simulink model "ArmDynamicsOnly"  (R2020a)
settings: Solver=FixedStepAuto  StartTime=0.0  StopTime=tsim  FixedStep=baseRate  MaxStep=0.0001  RelTol=1e-6  AbsTol=1e-6  EnableMultiTasking=on
values from neighbouring files (symbols this model uses):
  b0 = importdata("biases_layer_0.csv")    [Run_Initializer.m]
  b1 = importdata("biases_layer_1.csv")    [Run_Initializer.m]
  b_out = importdata("biases_output.csv")    [Run_Initializer.m]
  baseRate = 0.05    [Run_Initializer.m]
  CHASER_ABSOLUTE_POSITION = true    [Run_Initializer.m]
  drop_states_ARM = [ pi/2, pi/2, 0]    [Run_Initializer.m]
  drop_states_BLACK = [ xLength/2, yLength/2, pi]    [Run_Initializer.m]
  drop_states_BLUE = [ xLength/2, yLength/2, pi]    [Run_Initializer.m]
  drop_states_RED = [ xLength/2+0.5, yLength/2, pi]    [Run_Initializer.m]
  F_Black_X_nominal = 0.2196    [Run_Initializer.m]
  F_Black_Y_nominal = 0.2825    [Run_Initializer.m]
  F_Blue_X_nominal = 0.2196    [Run_Initializer.m]
  F_Blue_Y_nominal = 0.2825    [Run_Initializer.m]
  F_red_X_nominal = 0.2196    [Run_Initializer.m]
  F_red_Y_nominal = 0.2825    [Run_Initializer.m]
  F_thrusters_BLACK = [F_Black_X_nominal; F_Black_X_nominal;                             F_Black_Y_nominal; F_Black_Y_nominal; F_Black_X_nominal;                              F_Black_X_nominal; F_Black_Y_nominal; F_Black_Y_nominal]    [Run_Initializer.m]
  F_thrusters_BLUE = [F_Blue_X_nominal; F_Blue_X_nominal;                             F_Blue_Y_nominal; F_Blue_Y_nominal; F_Blue_X_nominal;                              F_Blue_X_nominal; F_Blue_Y_nominal; F_Blue_Y_nominal]    [Run_Initializer.m]
  F_thrusters_RED = [F_red_X_nominal; F_red_X_nominal;                             F_red_Y_nominal; F_red_Y_nominal; F_red_X_nominal;                              F_red_X_nominal; F_red_Y_nominal; F_red_Y_nominal]    [Run_Initializer.m]
  Gamma1_el = 0.12    [Run_Initializer.m]
  Gamma1_sh = 0.005    [Run_Initializer.m]
  Gamma1_wr = 0.025    [Run_Initializer.m]
  Gamma2_el = 5    [Run_Initializer.m]
  Gamma2_sh = 15    [Run_Initializer.m]
  Gamma2_wr = 5    [Run_Initializer.m]
  Gamma3_el = 10    [Run_Initializer.m]
  Gamma3_sh = 40    [Run_Initializer.m]
  Gamma3_wr = 40    [Run_Initializer.m]
  Gamma4_el = 0.039    [Run_Initializer.m]
  Gamma4_sh = 0.015    [Run_Initializer.m]
  Gamma4_wr = 0.029    [Run_Initializer.m]
  Gamma5_el = 800    [Run_Initializer.m]
  Gamma5_sh = 800    [Run_Initializer.m]
  Gamma5_wr = 800    [Run_Initializer.m]
  Gamma6_el = 0.000001    (= 1e-06)    [Run_Initializer.m]
  Gamma6_sh = 0.005    [Run_Initializer.m]
  Gamma6_wr = 0.02    [Run_Initializer.m]
  HOLD_POINT_RADIUS = 0.95    [Run_Initializer.m]
  home_states_BLACK = [ xLength/2; yLength/2; 0]    [Run_Initializer.m]
  home_states_BLUE = [ xLength/2; yLength/2; 0]    [Run_Initializer.m]
  home_states_RED = [ xLength/2+0.9; yLength/2; pi]    [Run_Initializer.m]
  init_states_BLACK = [ xLength/2; yLength/2; pi]    [Run_Initializer.m]
  init_states_BLUE = [ xLength/2; yLength/2; pi]    [Run_Initializer.m]
  init_states_RED = [ xLength/2+0.9; yLength/2; pi]    [Run_Initializer.m]
  Kd_tb = 1.0    (= 1)    [Run_Initializer.m]
  Kd_tblue = 1    [Run_Initializer.m]
  Kd_tr = 1.0    (= 1)    [Run_Initializer.m]
  Kd_xb = 8    [Run_Initializer.m]
  Kd_xblue = 8    [Run_Initializer.m]
  Kd_xr = 8    [Run_Initializer.m]
  Kd_yb = 8    [Run_Initializer.m]
  Kd_yblue = 8    [Run_Initializer.m]
  Kd_yr = 8    [Run_Initializer.m]
  Kp_tb = 0.1    [Run_Initializer.m]
  Kp_tblue = 0.1    [Run_Initializer.m]
  Kp_tr = 0.1    [Run_Initializer.m]
  Kp_xb = 2    [Run_Initializer.m]
  Kp_xblue = 2    [Run_Initializer.m]
  Kp_xr = 2    [Run_Initializer.m]
  Kp_yb = 2    [Run_Initializer.m]
  Kp_yblue = 2    [Run_Initializer.m]
  Kp_yr = 2    [Run_Initializer.m]
  MAX_BODY_ANGULAR_VELOCITY = 15*180/pi    (= 859.436692696)    [Run_Initializer.m]
  MAX_VELOCITY = 0.1    [Run_Initializer.m]
  noise_variance_BLACK = 0    [Run_Initializer.m]
  noise_variance_BLUE = 0    [Run_Initializer.m]
  noise_variance_RED = 0    [Run_Initializer.m]
  Phase0_End = Phase0_Duration    (= 10)    [Run_Initializer.m]
  Phase1_End = Phase0_Duration + Phase1_Duration    (= 15)    [Run_Initializer.m]
  Phase2_End = Phase0_Duration + Phase1_Duration +                                   Phase2_Duration    (= 45)    [Run_Initializer.m]
  Phase3_End = Phase0_Duration + Phase1_Duration +                                   Phase2_Duration + Phase3_Duration    (= 560)    [Run_Initializer.m]
  Phase3_SubPhase1_End = Phase2_End + Phase3_SubPhase1_Duration    (= 105)    [Run_Initializer.m]
  Phase3_SubPhase2_End = Phase2_End + Phase3_SubPhase1_Duration +                                   Phase3_SubPhase2_Duration    (= 210)    [Run_Initializer.m]
  Phase3_SubPhase3_End = Phase2_End + Phase3_SubPhase1_Duration +                                   Phase3_SubPhase2_Duration +                                  Phase3_SubPhase3_Duration    (= 240)    [Run_Initializer.m]
  Phase3_SubPhase4_End = Phase2_End + Phase3_SubPhase1_Duration +                                   Phase3_SubPhase2_Duration +                                  Phase3_SubPhase3_Duration +                                  Phase3_SubPhase4_Duration    [Run_Initializer.m]
  Phase4_End = Phase0_Duration + Phase1_Duration +                                   Phase2_Duration + Phase3_Duration +                                   Phase4_Duration    (= 680)    [Run_Initializer.m]
  Phase5_End = Phase0_Duration + Phase1_Duration +                                   Phase2_Duration + Phase3_Duration +                                   Phase4_Duration + Phase5_Duration    (= 700)    [Run_Initializer.m]
  relevant_half_range = (upper_state_bound - lower_state_bound)/2    [Run_Initializer.m]
  relevant_state_mean = (lower_state_bound + upper_state_bound)/2    [Run_Initializer.m]
  thruster_dist2CG_BLACK = [72.80;-65.20;61.75;-79.75;65.20;-65.20;74.25;-54.75]    [Run_Initializer.m]
  thruster_dist2CG_BLUE = [83.10;-54.90;71.50;-70.00;54.90;-75.50;64.50;-64.50]    [Run_Initializer.m]
  thruster_dist2CG_RED = [69.38;-56.62;50.01;-81.49;61.12;-68.38;78.99;-52.01]    [Run_Initializer.m]
  w0 = importdata("weights_layer_0.csv")    [Run_Initializer.m]
  w1 = importdata("weights_layer_1.csv")    [Run_Initializer.m]
  w_out = importdata("weights_output.csv")    [Run_Initializer.m]
  xLength = 3.51155    [Run_Initializer.m]
  yLength = 2.41935    [Run_Initializer.m]
undefined symbols (not defined in the file or in its folder): DiscIntNeverNeededParam, model_param, platformSelection, serverRate, simMode
libraries: dspstat3 x18, simulink x11, raspberrypiBasiclib x9, dspsigops x9, embdlinuxlib x7, MainLibrary x4, mspfiltlib x3, dsparch4 x3, etargetslib x1, sensehatlib x1
(part 12 of 14)

== matlab function ArmDynamicsOnly/Calculate Thruster ON//OFF/MATLAB Function7 ==
  data: H output; thruster_dist2CG_RED parameter; F_thrusters_RED parameter
function H = MakeH(thruster_dist2CG_RED,F_thrusters_RED)

Vec1 = [ -1
         -1
          0 
          0
          1
          1
          0
          0 ];
      
Vec2 = [  0
          0
          1
          1
          0
          0
         -1
         -1 ];
     
Vec3 = thruster_dist2CG_RED./1000;

Mat1 = [Vec1, Vec2, Vec3]';

Mat2 = diag((F_thrusters_RED./2));

H    = Mat1*Mat2;

end

== matlab function ArmDynamicsOnly/Calculate Thruster ON//OFF/MATLAB Function8 ==
  data: H output; thruster_dist2CG_RED parameter; F_red_X_nominal parameter; theta_1 input; theta_2 input; theta_3 input; model_param parameter; thrust_decay_factor input; F_red_Y_nominal parameter
function H   = MakeH(thruster_dist2CG_RED,F_red_X_nominal, theta_1, theta_2, theta_3, model_param, thrust_decay_factor, F_red_Y_nominal)


m0  = model_param(1);          
phi = model_param(7);
b0  = model_param(8);
a1  = model_param(9);
b1  = model_param(10);              
a2  = model_param(11);                
b2  = model_param(12);               
a3  = model_param(13);                         
m1  = model_param(15);
m2  = model_param(16);
m3  = model_param(17);

link1_com_x = b0*cos(phi) + a1*cos(pi/2 + theta_1);
link1_com_y = b0*sin(phi) + a1*sin(pi/2 + theta_1);

link2_com_x = link1_com_x + b1*cos(pi/2 + theta_1) + a2*cos(pi/2 + theta_1 + theta_2);
link2_com_y = link1_com_y + b1*sin(pi/2 + theta_1) + a2*sin(pi/2 + theta_1 + theta_2);

link3_com_x = link2_com_x + b2*cos(pi/2 + theta_1 + theta_2) + a3*cos(pi/2 + theta_1 + theta_2 + theta_3);
link3_com_y = link2_com_y + b2*sin(pi/2 + theta_1 + theta_2) + a3*sin(pi/2 + theta_1 + theta_2 + theta_3);

delta_com_due_to_arm_x = (m1*link1_com_x + m2*link2_com_x + m3*link3_com_x)/(m0 + m1 + m2 + m3)*1000; % [mm]
delta_com_due_to_arm_y = (m1*link1_com_y + m2*link2_com_y + m3*link3_com_y)/(m0 + m1 + m2 + m3)*1000; % [mm]

adjusted_thruster_dist2CG_RED = [thruster_dist2CG_RED(1)-delta_com_due_to_arm_y;
                                 thruster_dist2CG_RED(2)-delta_com_due_to_arm_y;
                                 thruster_dist2CG_RED(3)-delta_com_due_to_arm_x;
                                 thruster_dist2CG_RED(4)-delta_com_due_to_arm_x;
                                 thruster_dist2CG_RED(5)+delta_com_due_to_arm_y;
                                 thruster_dist2CG_RED(6)+delta_com_due_to_arm_y;
                                 thruster_dist2CG_RED(7)+delta_com_due_to_arm_x;
                                 thruster_dist2CG_RED(8)+delta_com_due_to_arm_x];
                                 


Vec1 = [ -1
         -1
          0 
          0
          1
          1
          0
          0 ];
      
Vec2 = [  0
          0
          1
          1
          0
          0
         -1
         -1 ];
     
Vec3 = adjusted_thruster_dist2CG_RED./1000;

Mat1 = [Vec1, Vec2, Vec3]';

F_thrusters_RED = [F_red_X_nominal*thrust_decay_factor; F_red_X_nominal*thrust_decay_factor; F_red_Y_nominal*thrust_decay_factor; F_red_Y_nominal*thrust_decay_factor; F_red_X_nominal*thrust_decay_factor; F_red_X_nominal*thrust_decay_factor; F_red_Y_nominal*thrust_decay_factor; F_red_Y_nominal*thrust_decay_factor];

Mat2 = diag((F_thrusters_RED));

H    = Mat1*Mat2;

end

== matlab function ArmDynamicsOnly/Calculate Thruster ON//OFF/MATLAB Function9 ==
  data: thrust_decay_factor output; PWMs input; thruster_count_threshold parameter; count output
function [thrust_decay_factor, count]  = check_thrust_decay(PWMs,thruster_count_threshold)

% normalize PWMs
if max(PWMs) > 1
    PWMs = PWMs/max(PWMs);
end

count = sum(PWMs > thruster_count_threshold);

positives_only = max(PWMs,0);
sum_of_duty_cycles = sum(positives_only);

average_duty_cycle_per_thruster = sum_of_duty_cycles/count;

% Look up the thrust decay for this average duty cycle
if (average_duty_cycle_per_thruster < 0.3) || (count == 0)
    thrust_decay_factor = 1;
else
    thrust_decay_factor = max(0.6 - 2*average_duty_cycle_per_thruster + 1, 0.5);   
end

== matlab function ArmDynamicsOnly/Calculate Thruster ON//OFF/Rotate Forces to Inertial1/Create Rotation Matrix ==
  data: Rz input; C_Ib output
function C_Ib = RotateFrame(Rz)

C_bI = [  cos(Rz) sin(Rz)
         -sin(Rz) cos(Rz) ];

C_Ib = inv(C_bI);

end

== matlab function ArmDynamicsOnly/Rotate Forces to Body/Create Rotation Matrix ==
  data: Rz input; C_bI output
function C_bI = RotateFrame(Rz)

C_bI = [  cos(Rz) sin(Rz)
         -sin(Rz) cos(Rz) ];

end

== matlab function ArmDynamicsOnly/Phase #5: Hold Home/Change RED Behavior/Hough Control/MATLAB Function2 ==
  data: Oy output; z input; Ox output
function [Oy, Ox]   = C3( z )
%C3 gives the rotation matrix about the z-axis for an angle 'z'
%   z - the angle about the z-axis which you rotate
%   A - the rotation matrix

Ox = [cos(z) sin(z); -sin(z) cos(z)]*[1;0];
Oy = [cos(z) sin(z); -sin(z) cos(z)]*[0;1];
end

== matlab function ArmDynamicsOnly/Phase #5: Hold Home/Change RED Behavior/Hough Control/MATLAB Function3 ==
  data: z input; Ox output
function Ox    = C3( z )
%C3 gives the rotation matrix about the z-axis for an angle 'z'
%   z - the angle about the z-axis which you rotate
%   A - the rotation matrix

Ox = [cos(z) sin(z); -sin(z) cos(z)]*[1;0];
end

== matlab function ArmDynamicsOnly/Phase #2: Move to Initial Position/Change BLACK Behavior/Hough Control/MATLAB Function3 ==
  data: z input; Ox output
function Ox    = C3( z )
%C3 gives the rotation matrix about the z-axis for an angle 'z'
%   z - the angle about the z-axis which you rotate
%   A - the rotation matrix

Ox = [cos(z) sin(z); -sin(z) cos(z)]*[1;0];
end

== matlab function ArmDynamicsOnly/Phase #5: Hold Home/Change RED Behavior/Hough Control/MATLAB Function4 ==
  data: Oy input; e_out output; e_in input
function e_out = fcn(Oy, e_in)

a = sign(Oy'*e_in);
e_out = -a*norm(e_in);

== matlab function ArmDynamicsOnly/From Force//Torque to PWM Signal/Change RED Behavior/Calculate Thruster ON//OFF/MATLAB Function10 ==
  data: H output; thruster_dist2CG_RED parameter; F_red_X_nominal parameter; theta_1 input; theta_2 input; theta_3 input; model_param parameter; thrust_decay_factor input; F_red_Y_nominal parameter
function H   = MakeHWithArmAndDecay(thruster_dist2CG_RED,F_red_X_nominal, theta_1, theta_2, theta_3, model_param, thrust_decay_factor, F_red_Y_nominal)

m0  = model_param(1);          
phi = model_param(7);
b0  = model_param(8);
a1  = model_param(9);
b1  = model_param(10);              
a2  = model_param(11);                
b2  = model_param(12);               
a3  = model_param(13);                         
m1  = model_param(15);
m2  = model_param(16);
m3  = model_param(17);

link1_com_x = b0*cos(phi) + a1*cos(pi/2 + theta_1);
link1_com_y = b0*sin(phi) + a1*sin(pi/2 + theta_1);

link2_com_x = link1_com_x + b1*cos(pi/2 + theta_1) + a2*cos(pi/2 + theta_1 + theta_2);
link2_com_y = link1_com_y + b1*sin(pi/2 + theta_1) + a2*sin(pi/2 + theta_1 + theta_2);

link3_com_x = link2_com_x + b2*cos(pi/2 + theta_1 + theta_2) + a3*cos(pi/2 + theta_1 + theta_2 + theta_3);
link3_com_y = link2_com_y + b2*sin(pi/2 + theta_1 + theta_2) + a3*sin(pi/2 + theta_1 + theta_2 + theta_3);

delta_com_due_to_arm_x = (m1*link1_com_x + m2*link2_com_x + m3*link3_com_x)/(m0 + m1 + m2 + m3)*1000; % [mm]
delta_com_due_to_arm_y = (m1*link1_com_y + m2*link2_com_y + m3*link3_com_y)/(m0 + m1 + m2 + m3)*1000; % [mm]

adjusted_thruster_dist2CG_RED = [thruster_dist2CG_RED(1)-delta_com_due_to_arm_y;
                                 thruster_dist2CG_RED(2)-delta_com_due_to_arm_y;
                                 thruster_dist2CG_RED(3)-delta_com_due_to_arm_x;
                                 thruster_dist2CG_RED(4)-delta_com_due_to_arm_x;
                                 thruster_dist2CG_RED(5)+delta_com_due_to_arm_y;
                                 thruster_dist2CG_RED(6)+delta_com_due_to_arm_y;
                                 thruster_dist2CG_RED(7)+delta_com_due_to_arm_x;
                                 thruster_dist2CG_RED(8)+delta_com_due_to_arm_x];
                                 


Vec1 = [ -1
         -1
          0 
          0
          1
          1
          0
          0 ];
      
Vec2 = [  0
          0
          1
          1
          0
          0
         -1
         -1 ];
     
Vec3 = adjusted_thruster_dist2CG_RED./1000;

Mat1 = [Vec1, Vec2, Vec3]';

F_thrusters_RED = [F_red_X_nominal*thrust_decay_factor; F_red_X_nominal*thrust_decay_factor; F_red_Y_nominal*thrust_decay_factor; F_red_Y_nominal*thrust_decay_factor; F_red_X_nominal*thrust_decay_factor; F_red_X_nominal*thrust_decay_factor; F_red_Y_nominal*thrust_decay_factor; F_red_Y_nominal*thrust_decay_factor];

Mat2 = diag((F_thrusters_RED./2));

H    = Mat1*Mat2;

end

== matlab function ArmDynamicsOnly/From Force//Torque to PWM Signal/Change RED Behavior/Calculate Thruster ON//OFF/MATLAB Function3 ==
  data: H output; thruster_dist2CG_RED parameter; F_thrusters_RED parameter; theta_1 input; theta_2 input; theta_3 input; model_param parameter
function H   = MakeHWithArm(thruster_dist2CG_RED,F_thrusters_RED, theta_1, theta_2, theta_3, model_param)

m0  = model_param(1);          
phi = model_param(7);
b0  = model_param(8);
a1  = model_param(9);
b1  = model_param(10);              
a2  = model_param(11);                
b2  = model_param(12);               
a3  = model_param(13);                         
m1  = model_param(15);
m2  = model_param(16);
m3  = model_param(17);

link1_com_x = b0*cos(phi) + a1*cos(pi/2 + theta_1);
link1_com_y = b0*sin(phi) + a1*sin(pi/2 + theta_1);

link2_com_x = link1_com_x + b1*cos(pi/2 + theta_1) + a2*cos(pi/2 + theta_1 + theta_2);
link2_com_y = link1_com_y + b1*sin(pi/2 + theta_1) + a2*sin(pi/2 + theta_1 + theta_2);

link3_com_x = link2_com_x + b2*cos(pi/2 + theta_1 + theta_2) + a3*cos(pi/2 + theta_1 + theta_2 + theta_3);
link3_com_y = link2_com_y + b2*sin(pi/2 + theta_1 + theta_2) + a3*sin(pi/2 + theta_1 + theta_2 + theta_3);

delta_com_due_to_arm_x = (m1*link1_com_x + m2*link2_com_x + m3*link3_com_x)/(m0 + m1 + m2 + m3)*1000; % [mm]
delta_com_due_to_arm_y = (m1*link1_com_y + m2*link2_com_y + m3*link3_com_y)/(m0 + m1 + m2 + m3)*1000; % [mm]

adjusted_thruster_dist2CG_RED = [thruster_dist2CG_RED(1)-delta_com_due_to_arm_y;
                                 thruster_dist2CG_RED(2)-delta_com_due_to_arm_y;
                                 thruster_dist2CG_RED(3)-delta_com_due_to_arm_x;
                                 thruster_dist2CG_RED(4)-delta_com_due_to_arm_x;
                                 thruster_dist2CG_RED(5)+delta_com_due_to_arm_y;
                                 thruster_dist2CG_RED(6)+delta_com_due_to_arm_y;
                                 thruster_dist2CG_RED(7)+delta_com_due_to_arm_x;
                                 thruster_dist2CG_RED(8)+delta_com_due_to_arm_x];
                                 


Vec1 = [ -1
         -1
          0 
          0
          1
          1
          0
          0 ];
      
Vec2 = [  0
          0
          1
          1
          0
          0
         -1
         -1 ];
     
Vec3 = adjusted_thruster_dist2CG_RED./1000;

Mat1 = [Vec1, Vec2, Vec3]';

Mat2 = diag((F_thrusters_RED./2));

H    = Mat1*Mat2;

end

== matlab function ArmDynamicsOnly/From Force//Torque to PWM Signal/Change RED Behavior/Calculate Thruster ON//OFF/MATLAB Function4 ==
  data: H output; thruster_dist2CG_RED parameter; F_thrusters_RED parameter
function H = MakeH(thruster_dist2CG_RED,F_thrusters_RED)

Vec1 = [ -1
         -1
          0 
          0
          1
          1
          0
          0 ];
      
Vec2 = [  0
          0
          1
          1
          0
          0
         -1
         -1 ];
     
Vec3 = thruster_dist2CG_RED./1000;

Mat1 = [Vec1, Vec2, Vec3]';

Mat2 = diag((F_thrusters_RED));

H    = Mat1*Mat2;

end

== matlab function ArmDynamicsOnly/From Force//Torque to PWM Signal/Change RED Behavior/Calculate Thruster ON//OFF/MATLAB Function6 ==
  data: ThrustPer_Final output; ThrustPer input
function ThrustPer_Final  = ThrusterSat(ThrustPer)

ValveTime       = 0.007;
TControl        = 0.1;
ThrustPer_Final = zeros(8,1);

if max(ThrustPer) > 1
    ThrustPer_Sat = ThrustPer/max(ThrustPer);
else
    ThrustPer_Sat = ThrustPer;
end

for i = 1:8
    if ThrustPer_Sat(i) > ValveTime/TControl 
        ThrustPer_Final(i) = ThrustPer_Sat(i);
    else
        ThrustPer_Final(i) = 0;
    end
end
   

end

== matlab function ArmDynamicsOnly/From Force//Torque to PWM Signal/Change RED Behavior/Calculate Thruster ON//OFF/MATLAB Function7 ==
  data: H output; thruster_dist2CG_RED parameter; F_thrusters_RED parameter
function H = MakeH(thruster_dist2CG_RED,F_thrusters_RED)

Vec1 = [ -1
         -1
          0 
          0
          1
          1
          0
          0 ];
      
Vec2 = [  0
          0
          1
          1
          0
          0
         -1
         -1 ];
     
Vec3 = thruster_dist2CG_RED./1000;

Mat1 = [Vec1, Vec2, Vec3]';

Mat2 = diag((F_thrusters_RED./2));

H    = Mat1*Mat2;

end

== matlab function ArmDynamicsOnly/From Force//Torque to PWM Signal/Change RED Behavior/Calculate Thruster ON//OFF/MATLAB Function8 ==
  data: H output; thruster_dist2CG_RED parameter; F_red_X_nominal parameter; theta_1 input; theta_2 input; theta_3 input; model_param parameter; thrust_decay_factor input; F_red_Y_nominal parameter
function H   = MakeH(thruster_dist2CG_RED,F_red_X_nominal, theta_1, theta_2, theta_3, model_param, thrust_decay_factor, F_red_Y_nominal)


m0  = model_param(1);          
phi = model_param(7);
b0  = model_param(8);
a1  = model_param(9);
b1  = model_param(10);              
a2  = model_param(11);                
b2  = model_param(12);               
a3  = model_param(13);                         
m1  = model_param(15);
m2  = model_param(16);
m3  = model_param(17);

link1_com_x = b0*cos(phi) + a1*cos(pi/2 + theta_1);
link1_com_y = b0*sin(phi) + a1*sin(pi/2 + theta_1);

link2_com_x = link1_com_x + b1*cos(pi/2 + theta_1) + a2*cos(pi/2 + theta_1 + theta_2);
link2_com_y = link1_com_y + b1*sin(pi/2 + theta_1) + a2*sin(pi/2 + theta_1 + theta_2);

link3_com_x = link2_com_x + b2*cos(pi/2 + theta_1 + theta_2) + a3*cos(pi/2 + theta_1 + theta_2 + theta_3);
link3_com_y = link2_com_y + b2*sin(pi/2 + theta_1 + theta_2) + a3*sin(pi/2 + theta_1 + theta_2 + theta_3);

delta_com_due_to_arm_x = (m1*link1_com_x + m2*link2_com_x + m3*link3_com_x)/(m0 + m1 + m2 + m3)*1000; % [mm]
delta_com_due_to_arm_y = (m1*link1_com_y + m2*link2_com_y + m3*link3_com_y)/(m0 + m1 + m2 + m3)*1000; % [mm]

adjusted_thruster_dist2CG_RED = [thruster_dist2CG_RED(1)-delta_com_due_to_arm_y;
                                 thruster_dist2CG_RED(2)-delta_com_due_to_arm_y;
                                 thruster_dist2CG_RED(3)-delta_com_due_to_arm_x;
                                 thruster_dist2CG_RED(4)-delta_com_due_to_arm_x;
                                 thruster_dist2CG_RED(5)+delta_com_due_to_arm_y;
                                 thruster_dist2CG_RED(6)+delta_com_due_to_arm_y;
                                 thruster_dist2CG_RED(7)+delta_com_due_to_arm_x;
                                 thruster_dist2CG_RED(8)+delta_com_due_to_arm_x];
                                 


Vec1 = [ -1
         -1
          0 
          0
          1
          1
          0
          0 ];
      
Vec2 = [  0
          0
          1
          1
          0
          0
         -1
         -1 ];
     
Vec3 = adjusted_thruster_dist2CG_RED./1000;

Mat1 = [Vec1, Vec2, Vec3]';

F_thrusters_RED = [F_red_X_nominal*thrust_decay_factor; F_red_X_nominal*thrust_decay_factor; F_red_Y_nominal*thrust_decay_factor; F_red_Y_nominal*thrust_decay_factor; F_red_X_nominal*thrust_decay_factor; F_red_X_nominal*thrust_decay_factor; F_red_Y_nominal*thrust_decay_factor; F_red_Y_nominal*thrust_decay_factor];

Mat2 = diag((F_thrusters_RED));

H    = Mat1*Mat2;

end

== matlab function ArmDynamicsOnly/Phase #2: Move to Initial Position/Change BLACK Behavior/Hough Control/MATLAB Function4 ==
  data: Oy input; e_out output; e_in input
function e_out = fcn(Oy, e_in)

a = sign(Oy'*e_in);
e_out = -a*norm(e_in);

== matlab function ArmDynamicsOnly/From Force//Torque to PWM Signal/Change RED Behavior/Calculate Thruster ON//OFF/MATLAB Function9 ==
  data: thrust_decay_factor output; PWMs input; thruster_count_threshold parameter; count output
function [thrust_decay_factor, count]  = check_thrust_decay(PWMs,thruster_count_threshold)

% normalize PWMs
if max(PWMs) > 1
    PWMs = PWMs/max(PWMs);
end

count = sum(PWMs > thruster_count_threshold);

positives_only = max(PWMs,0);
sum_of_duty_cycles = sum(positives_only);

average_duty_cycle_per_thruster = sum_of_duty_cycles/count;

% Look up the thrust decay for this average duty cycle
if (average_duty_cycle_per_thruster < 0.3) || (count == 0)
    thrust_decay_factor = 1;
else
    thrust_decay_factor = max(0.6 - 2*average_duty_cycle_per_thruster + 1, 0.5);   
end

== matlab function ArmDynamicsOnly/From Force//Torque to PWM Signal/Change RED Behavior/Calculate Thruster ON//OFF/Rotate Forces to Inertial1/Create Rotation Matrix ==
  data: Rz input; C_Ib output
function C_Ib = RotateFrame(Rz)

C_bI = [  cos(Rz) sin(Rz)
         -sin(Rz) cos(Rz) ];

C_Ib = inv(C_bI);

end

== matlab function ArmDynamicsOnly/From Force//Torque to PWM Signal/Change BLACK Behavior/Calculate Thruster ON//OFF/MATLAB Function ==
  data: H output; thruster_dist2CG_BLACK parameter; F_thrusters_BLACK parameter
function H = MakeH(thruster_dist2CG_BLACK,F_thrusters_BLACK)

Vec1 = [ -1
         -1
          0 
          0
          1
          1
          0
          0 ];
      
Vec2 = [  0
          0
          1
          1
          0
          0
         -1
         -1 ];
     
Vec3 = thruster_dist2CG_BLACK./1000;

Mat1 = [Vec1, Vec2, Vec3]';

Mat2 = diag((F_thrusters_BLACK./2));

H    = Mat1*Mat2;

end

== matlab function ArmDynamicsOnly/Phase #3: Experiment/Change BLACK Behavior/Sub-Phase #4/BLACK_RzD/Wrap1/MATLAB Function ==
  data: u input; wrappedAngle output
function wrappedAngle = wrapAngle(u)

wrappedAngle = atan2(sin(u),cos(u));

end

== matlab function ArmDynamicsOnly/Phase #3: Experiment/Change BLACK Behavior/Sub-Phase #2 /BLACK_RzD1/Wrap1/MATLAB Function ==
  data: u input; wrappedAngle output
function wrappedAngle = wrapAngle(u)

wrappedAngle = atan2(sin(u),cos(u));

end

== matlab function ArmDynamicsOnly/From Force//Torque to PWM Signal/Change BLACK Behavior/Calculate Thruster ON//OFF/MATLAB Function1 ==
  data: H output; thruster_dist2CG_BLACK parameter; F_thrusters_BLACK parameter
function H = MakeH(thruster_dist2CG_BLACK,F_thrusters_BLACK)

Vec1 = [ -1
         -1
          0 
          0
          1
          1
          0
          0 ];
      
Vec2 = [  0
          0
          1
          1
          0
          0
         -1
         -1 ];
     
Vec3 = thruster_dist2CG_BLACK./1000;

Mat1 = [Vec1, Vec2, Vec3]';

Mat2 = diag((F_thrusters_BLACK));

H    = Mat1*Mat2;

end

== matlab function ArmDynamicsOnly/From Force//Torque to PWM Signal/Change BLACK Behavior/Calculate Thruster ON//OFF/MATLAB Function2 ==
  data: ThrustPer_Final output; ThrustPer input
function ThrustPer_Final  = ThrusterSat(ThrustPer)

ValveTime       = 0.007;
TControl        = 0.1;
ThrustPer_Final = zeros(8,1);

if max(ThrustPer) > 1
    ThrustPer_Sat = ThrustPer/max(ThrustPer);
else
    ThrustPer_Sat = ThrustPer;
end

for i = 1:8
    if ThrustPer_Sat(i) > ValveTime/TControl 
        ThrustPer_Final(i) = ThrustPer_Sat(i);
    else
        ThrustPer_Final(i) = 0;
    end
end
   

end

== matlab function ArmDynamicsOnly/From Force//Torque to PWM Signal/Change BLACK Behavior/Calculate Thruster ON//OFF/Rotate Forces to Inertial/Create Rotation Matrix ==
  data: Rz input; C_Ib output
function C_Ib = RotateFrame(Rz)

C_bI = [  cos(Rz) sin(Rz)
         -sin(Rz) cos(Rz) ];

C_Ib = inv(C_bI);

end

== matlab function ArmDynamicsOnly/From Force//Torque to PWM Signal/Change BLACK Behavior/Rotate Forces to Body/Create Rotation Matrix ==
  data: Rz input; C_bI output
function C_bI = RotateFrame(Rz)

C_bI = [  cos(Rz) sin(Rz)
         -sin(Rz) cos(Rz) ];

end

== matlab function ArmDynamicsOnly/Phase #3: Experiment/Change RED Behavior/Sub-Phase #2 /Hough Control/MATLAB Function2 ==
  data: Oy output; z input; Ox output
function [Oy, Ox]   = C3( z )
%C3 gives the rotation matrix about the z-axis for an angle 'z'
%   z - the angle about the z-axis which you rotate
%   A - the rotation matrix

Ox = [cos(z) sin(z); -sin(z) cos(z)]*[1;0];
Oy = [cos(z) sin(z); -sin(z) cos(z)]*[0;1];
end

== matlab function ArmDynamicsOnly/Phase #3: Experiment/Change RED Behavior/Sub-Phase #3 /Hough Control/MATLAB Function2 ==
  data: Oy output; z input; Ox output
function [Oy, Ox]   = C3( z )
%C3 gives the rotation matrix about the z-axis for an angle 'z'
%   z - the angle about the z-axis which you rotate
%   A - the rotation matrix

Ox = [cos(z) sin(z); -sin(z) cos(z)]*[1;0];
Oy = [cos(z) sin(z); -sin(z) cos(z)]*[0;1];
end

== matlab function ArmDynamicsOnly/Phase #3: Experiment/Change RED Behavior/Sub-Phase #4/calculate_mass_matrix ==
  data: M output
function M  = generate_M()
  
    m0                 = 13.80;     % RED Mass
    I0                = 0.242150;      % RED Inertia;
   


    M = [m0 0 0
         0 m0 0
         0 0 I0];

end
% Artificially setting M_31 and M_32 to zero, such that the feedforward
% controller does not think a torque needs to be applied to the base to
% counteract the torque needed to maintain the angular acceleration of the
% links when the base has a linear acceleration. No torque is applied to keep the links at their linear
% acceleration because friction does this for us.

% The original matrix
% M = reshape([t17,0.0,t30,-t86-t87-t88,-t88-t13.*t28,-t88,...
%     0.0,t17,t33,-t89-t90-t91,-t91-t24.*t28,-t91,...
%     t30,t33,...
%     I0+I1+I2+I3+t46+t51+t57+t64+t65+t66+t67+t68+t70+t71+t72+t74+t75+t76+t77+t59.*(a1.*b0.*m1.*2.0+a1.*b0.*m2.*2.0+a1.*b0.*m3.*2.0+b0.*b1.*m2.*2.0+b0.*b1.*m3.*2.0)+m1.*t36+m2.*t36+m3.*t36-t61.*(a2.*b0.*m2.*2.0+a2.*b0.*m3.*2.0+b0.*b2.*m3.*2.0)-a3.*b0.*m3.*t63.*2.0,t99,I2+I3+t51+t67+t68+t70+t74+t77+t85+t107-t112-t113,I3+t70+t85+t111-t113,-t7.*t8-t13.*t14-a3.*m3.*t16,    -t8.*t23-t14.*t24-a3.*m3.*t25,t99,I1+I2+I3+t46+t51+t57+t64+t65+t66+t67+t68+t70+t71+t72+t74+t75+t76+t77,t114,t115,-t13.*t28-a3.*m3.*t16,-t24.*t28-a3.*m3.*t25,I2+I3+t51+t67+t68+t70+t74+t77+t85+t107-t61.*t81-a3.*b0.*m3.*t63,t114,I2+I3+t51+t67+t68+t70+t74+t77,t116,-a3.*m3.*t16,-a3.*m3.*t25,I3+t70+t85+t111-a3.*b0.*m3.*t63,t115,t116,I3+t70],[6,6]);

== matlab function ArmDynamicsOnly/Phase #3: Experiment/Change RED Behavior/Sub-Phase #4/RED+ARM/Transpose Jacobian Controller/Arm Controller/MATLAB Function ==
  data: dx input; dxd input; dxi input; TAU output; qdot input; Jt input
function TAU  = fcn(dx, dxd, dxi, qdot, Jt)
%#codegen

Kp = [1500 0 0
      0    1500 0
      0    0    1500];
Kv = [50 0 0
      0    50 0
      0    0    50];    
Ki = [200 0 0
      0    200 0
      0    0    200]; 
% Source: http://ieeexplore.ieee.org.proxy.library.carleton.ca/stamp/stamp.jsp?tp=&arnumber=34766
q1_d   = qdot(1);
q2_d   = qdot(2);
q3_d   = qdot(3);

% Control Law
TAU = Kp*Jt*dx' + Kv*Jt*dxd' + Ki*Jt*dxi';% + Kv*[ q1_d q2_d q3_d];
                   

end

== matlab function ArmDynamicsOnly/Simulate Plant Dynamics/RED and ARM Dynamics/RED Only/RED Dynamics/Sample and Hold Data to Match PhaseSpace (RED)/MATLAB Function ==
  data: TIME input; y output; SERVER input
function y = fcn(TIME, SERVER)

if mod(TIME,SERVER) == 0
    y = 1;
else
    y = 0;
end

== matlab function ArmDynamicsOnly/Simulate Plant Dynamics/BLACK Dynamics/Sample and Hold Data to Match PhaseSpace (BLACK)/MATLAB Function ==
  data: TIME input; y output; SERVER input
function y = fcn(TIME, SERVER)

if mod(TIME,SERVER) == 0
    y = 1;
else
    y = 0;
end

== matlab function ArmDynamicsOnly/From Force//Torque to PWM Signal/Change RED Behavior/Rotate Forces to Body/Create Rotation Matrix ==
  data: Rz input; C_bI output
function C_bI = RotateFrame(Rz)

C_bI = [  cos(Rz) sin(Rz)
         -sin(Rz) cos(Rz) ];

end

== matlab function ArmDynamicsOnly/Phase #2: Move to Initial Position/Change RED Behavior/Hough Control/MATLAB Function2 ==
  data: Oy output; z input; Ox output
function [Oy, Ox]   = C3( z )
%C3 gives the rotation matrix about the z-axis for an angle 'z'
%   z - the angle about the z-axis which you rotate
%   A - the rotation matrix

Ox = [cos(z) sin(z); -sin(z) cos(z)]*[1;0];
Oy = [cos(z) sin(z); -sin(z) cos(z)]*[0;1];
end

== matlab function ArmDynamicsOnly/Phase #2: Move to Initial Position/Change RED Behavior/Hough Control/MATLAB Function3 ==
  data: z input; Ox output
function Ox    = C3( z )
%C3 gives the rotation matrix about the z-axis for an angle 'z'
%   z - the angle about the z-axis which you rotate
%   A - the rotation matrix

Ox = [cos(z) sin(z); -sin(z) cos(z)]*[1;0];
end

== matlab function ArmDynamicsOnly/Phase #2: Move to Initial Position/Change RED Behavior/Hough Control/MATLAB Function4 ==
  data: Oy input; e_out output; e_in input
function e_out = fcn(Oy, e_in)

a = sign(Oy'*e_in);
e_out = -a*norm(e_in);

== matlab function ArmDynamicsOnly/Phase #3: Experiment/Change BLACK Behavior/Sub-Phase #2 /Hough Control/MATLAB Function2 ==
  data: Oy output; z input; Ox output
function [Oy, Ox]   = C3( z )
%C3 gives the rotation matrix about the z-axis for an angle 'z'
%   z - the angle about the z-axis which you rotate
%   A - the rotation matrix

Ox = [cos(z) sin(z); -sin(z) cos(z)]*[1;0];
Oy = [cos(z) sin(z); -sin(z) cos(z)]*[0;1];
end

== matlab function ArmDynamicsOnly/Phase #4: Return Home/Change BLACK Behavior/Hough Control/MATLAB Function2 ==
  data: Oy output; z input; Ox output
function [Oy, Ox]   = C3( z )
%C3 gives the rotation matrix about the z-axis for an angle 'z'
%   z - the angle about the z-axis which you rotate
%   A - the rotation matrix

Ox = [cos(z) sin(z); -sin(z) cos(z)]*[1;0];
Oy = [cos(z) sin(z); -sin(z) cos(z)]*[0;1];
end

== matlab function ArmDynamicsOnly/Phase #4: Return Home/Change BLACK Behavior/Hough Control/MATLAB Function3 ==
  data: z input; Ox output
function Ox    = C3( z )
%C3 gives the rotation matrix about the z-axis for an angle 'z'
%   z - the angle about the z-axis which you rotate
%   A - the rotation matrix

Ox = [cos(z) sin(z); -sin(z) cos(z)]*[1;0];
end

== matlab function ArmDynamicsOnly/Phase #4: Return Home/Change BLACK Behavior/Hough Control/MATLAB Function4 ==
  data: Oy input; e_out output; e_in input
function e_out = fcn(Oy, e_in)

a = sign(Oy'*e_in);
e_out = -a*norm(e_in);

== matlab function ArmDynamicsOnly/Phase #4: Return Home/Change RED Behavior/Hough Control/MATLAB Function2 ==
  data: Oy output; z input; Ox output
function [Oy, Ox]   = C3( z )
%C3 gives the rotation matrix about the z-axis for an angle 'z'
%   z - the angle about the z-axis which you rotate
%   A - the rotation matrix

Ox = [cos(z) sin(z); -sin(z) cos(z)]*[1;0];
Oy = [cos(z) sin(z); -sin(z) cos(z)]*[0;1];
end

== matlab function ArmDynamicsOnly/Phase #4: Return Home/Change RED Behavior/Hough Control/MATLAB Function3 ==
  data: z input; Ox output
function Ox    = C3( z )
%C3 gives the rotation matrix about the z-axis for an angle 'z'
%   z - the angle about the z-axis which you rotate
%   A - the rotation matrix

Ox = [cos(z) sin(z); -sin(z) cos(z)]*[1;0];
end

== matlab function ArmDynamicsOnly/Phase #4: Return Home/Change RED Behavior/Hough Control/MATLAB Function4 ==
  data: Oy input; e_out output; e_in input
function e_out = fcn(Oy, e_in)

a = sign(Oy'*e_in);
e_out = -a*norm(e_in);

== matlab function ArmDynamicsOnly/Phase #2: Move to Initial Position/Change BLUE Behavior/Hough Control/MATLAB Function2 ==
  data: Oy output; z input; Ox output
function [Oy, Ox]   = C3( z )
%C3 gives the rotation matrix about the z-axis for an angle 'z'
%   z - the angle about the z-axis which you rotate
%   A - the rotation matrix

Ox = [cos(z) sin(z); -sin(z) cos(z)]*[1;0];
Oy = [cos(z) sin(z); -sin(z) cos(z)]*[0;1];
end

== matlab function ArmDynamicsOnly/Phase #2: Move to Initial Position/Change BLUE Behavior/Hough Control/MATLAB Function3 ==
  data: z input; Ox output
function Ox    = C3( z )
%C3 gives the rotation matrix about the z-axis for an angle 'z'
%   z - the angle about the z-axis which you rotate
%   A - the rotation matrix

Ox = [cos(z) sin(z); -sin(z) cos(z)]*[1;0];
end

== matlab function ArmDynamicsOnly/Phase #2: Move to Initial Position/Change BLUE Behavior/Hough Control/MATLAB Function4 ==
  data: Oy input; e_out output; e_in input
function e_out = fcn(Oy, e_in)

a = sign(Oy'*e_in);
e_out = -a*norm(e_in);

== matlab function ArmDynamicsOnly/Phase #3: Experiment/Change BLUE Behavior/Sub-Phase #1/BLACK_RzD1/Wrap1/MATLAB Function ==
  data: u input; wrappedAngle output
function wrappedAngle = wrapAngle(u)

wrappedAngle = atan2(sin(u),cos(u));

end

== matlab function ArmDynamicsOnly/Phase #3: Experiment/Change BLACK Behavior/Sub-Phase #2 /Hough Control/MATLAB Function3 ==
  data: z input; Ox output
function Ox    = C3( z )
%C3 gives the rotation matrix about the z-axis for an angle 'z'
%   z - the angle about the z-axis which you rotate
%   A - the rotation matrix

Ox = [cos(z) sin(z); -sin(z) cos(z)]*[1;0];
end

== matlab function ArmDynamicsOnly/Phase #3: Experiment/Change RED Behavior/Sub-Phase #1/Hough Control/MATLAB Function2 ==
  data: Oy output; z input; Ox output
function [Oy, Ox]   = C3( z )
%C3 gives the rotation matrix about the z-axis for an angle 'z'
%   z - the angle about the z-axis which you rotate
%   A - the rotation matrix

Ox = [cos(z) sin(z); -sin(z) cos(z)]*[1;0];
Oy = [cos(z) sin(z); -sin(z) cos(z)]*[0;1];
end

== matlab function ArmDynamicsOnly/Phase #3: Experiment/Change BLACK Behavior/Sub-Phase #2 /Hough Control/MATLAB Function4 ==
  data: Oy input; e_out output; e_in input
function e_out = fcn(Oy, e_in)

a = sign(Oy'*e_in);
e_out = -a*norm(e_in);

== matlab function ArmDynamicsOnly/Phase #3: Experiment/Change BLUE Behavior/Sub-Phase #1/Hough Control/MATLAB Function2 ==
  data: Oy output; z input; Ox output
function [Oy, Ox]   = C3( z )
%C3 gives the rotation matrix about the z-axis for an angle 'z'
%   z - the angle about the z-axis which you rotate
%   A - the rotation matrix

Ox = [cos(z) sin(z); -sin(z) cos(z)]*[1;0];
Oy = [cos(z) sin(z); -sin(z) cos(z)]*[0;1];
end

== matlab function ArmDynamicsOnly/Phase #3: Experiment/Change BLUE Behavior/Sub-Phase #1/Hough Control/MATLAB Function3 ==
  data: z input; Ox output
function Ox    = C3( z )
%C3 gives the rotation matrix about the z-axis for an angle 'z'
%   z - the angle about the z-axis which you rotate
%   A - the rotation matrix

Ox = [cos(z) sin(z); -sin(z) cos(z)]*[1;0];
end

== matlab function ArmDynamicsOnly/Phase #3: Experiment/Change BLUE Behavior/Sub-Phase #4/BLACK_RzD1/Wrap1/MATLAB Function ==
  data: u input; wrappedAngle output
function wrappedAngle = wrapAngle(u)

wrappedAngle = atan2(sin(u),cos(u));

end

== matlab function ArmDynamicsOnly/Phase #3: Experiment/Change BLACK Behavior/Sub-Phase #3 /BLACK_RzD1/Wrap1/MATLAB Function ==
  data: u input; wrappedAngle output
function wrappedAngle = wrapAngle(u)

wrappedAngle = atan2(sin(u),cos(u));

end

== matlab function ArmDynamicsOnly/Jetson Communication/Kirk Network Control (SIM)/MATLAB Function ==
  data: Pi_time input; Ax_command output; Pi_red_x input; Pi_red_y input; Pi_red_theta input; Pi_red_Vx input; Pi_red_Vy input; Pi_red_omega input; Pi_black_x input; Pi_black_y input; Pi_black_theta input; Pi_black_Vx input; Pi_black_Vy input; Pi_black_omega input; Ay_command output; Az_command output; CHASER_ABSOLUTE_POSITION parameter; relevant_state_mean parameter; relevant_half_range parameter; w0 parameter; b0 parameter; w1 parameter; b1 parameter; w_out parameter; b_out parameter; MAX_VELOCITY parameter; MAX_BODY_ANGULAR_VELOCITY parameter; HOLD_POINT_RADIUS input; control_inputs input; vx_prev input; vy_prev input; omega_prev input; model_param parameter
function [Ax_command, Ay_command, Az_command] = guidance_server_sim(Pi_time, Pi_red_x, Pi_red_y, Pi_red_theta, Pi_red_Vx, Pi_red_Vy,...
                                 Pi_red_omega, Pi_black_x, Pi_black_y, Pi_black_theta, Pi_black_Vx,...
                                 Pi_black_Vy, Pi_black_omega, CHASER_ABSOLUTE_POSITION, relevant_state_mean, relevant_half_range, w0, b0, w1, b1, w_out, b_out, MAX_VELOCITY,...
                                 MAX_BODY_ANGULAR_VELOCITY, HOLD_POINT_RADIUS, control_inputs, vx_prev, vy_prev, omega_prev,...
model_param)
    % For testing
    SPOTNet_sees_target = false;
    VELOCITY_LIMIT = [MAX_VELOCITY, MAX_VELOCITY,MAX_BODY_ANGULAR_VELOCITY]; 
    
    
    if SPOTNet_sees_target == true
        
        % Insert logic that uses the vision data
        
        output = [0,0,0];
        
    else
        
        % Use a basic model to predict where the target is more likely to
        % be:
       
        % Extract the servicer model parameters from the model_param vector defined
        % in initialize.m:
        m_BLACK    = model_param(3);
        I_BLACK    = model_param(4);

        % Extract the control inputs from the control_input vector:
        Fx        = control_inputs(1);              % [N]
        Fy        = control_inputs(2);              % [N]
        Tz        = control_inputs(3);              % [N.m]

        % Calculate the state acceleration vector:
        ax_pred    = Fx/m_BLACK;                      % [m/s^2]
        ay_pred    = Fy/m_BLACK;                      % [m/s^2]
        alpha_pred = Tz/I_BLACK;                      % [rad/s^2]
        
        vx_pred = vx_prev + ax_pred*0.48;
        vy_pred = vy_prev + ay_pred*0.48;
        omega_pred = omega_prev + alpha_pred*0.48;
        
        px_pred = Pi_black_x + vx_pred*0.48;
        py_pred = Pi_black_y + vy_pred*0.48;
        theta_pred = Pi_black_theta + omega_pred*0.48;
               
        % We don't see the target -> Use PhaseSpace only
        % Calculating the relative X and Y in the chaser's body frame using PhaseSpace
        %relative_pose_inertial = [Pi_black_x - Pi_red_x, Pi_black_y - Pi_red_y, Pi_black_theta - Pi_red_theta];
        relative_pose_inertial = [px_pred - Pi_red_x, py_pred - Pi_red_y,theta_pred - Pi_red_theta];
        
        % Calculate the roation matrix from inertia to body
        C_bI_red = [ cos(Pi_red_theta), sin(Pi_red_theta);...
                -sin(Pi_red_theta), cos(Pi_red_theta)];
        
        % Calculate relative body pose    
        %relative_pose_body     = C_bI_red*relative_pose_inertial;
        
        % With chaser absolute position
        % policy_input = np.array([relative_pose_body[0] - self.offset_x, relative_pose_body[1] - self.offset_y, (self.SPOTNet_target_angle_inertial - Pi_red_theta - self.offset_angle)%(2*np.pi), Pi_red_x, Pi_red_y, Pi_red_theta, Pi_red_Vx, Pi_red_Vy, Pi_red_omega, Pi_black_omega])

        %############# New policy input as of Nov 9 2022                    
        % Calculate the desired X, Y, theta, Vx, Vy, omega 
        % relative to the chaser's current state
        % all in the inertial frame                 

        %Calculate desired position and velocity in the inertial frame
        desired_position_relative_to_target_I = [-sin(Pi_black_theta)*(HOLD_POINT_RADIUS), cos(Pi_black_theta)*(HOLD_POINT_RADIUS), -pi/2];
        desired_position_I = [Pi_black_x, Pi_black_y, Pi_black_theta] + desired_position_relative_to_target_I;
        desired_velocity_I = [Pi_black_Vx, Pi_black_Vy, Pi_black_omega] + cross([0,0,Pi_black_omega], desired_position_relative_to_target_I);

        % Now calculate the chaser's relative position and velocity to that desired location and velocity in the inertial frame
        chaser_position_error_inertial = desired_position_I - [Pi_red_x, Pi_red_y, Pi_red_theta];
        chaser_velocity_error_inertial = desired_velocity_I - [Pi_red_Vx, Pi_red_Vy, Pi_red_omega];
        policy_input = [Pi_red_x, Pi_red_y, mod(Pi_red_theta, 2*pi), Pi_red_Vx, Pi_red_Vy, Pi_red_omega, relative_pose_inertial, chaser_position_error_inertial, chaser_velocity_error_inertial];

        % Normalize the states
        normalized_policy_input = (policy_input - relevant_state_mean)./relevant_half_range;
        
        % Run the policy input through the neural network
        
        % First fully-connected layer
        layer_1 = max(0,normalized_policy_input*w0 + b0);

        % Second fully-connected layer
        layer_2 = max(0,layer_1*w1 + b1);

        % Output layer
        output = tanh(layer_2*w_out + b_out);
        
        % Convert commands
        output(1) = output(1).*0.01;
        output(2) = output(2).*0.01;
        output(3) = output(3).*0.02;
        
        % Transform back to inertial
        %output(1:2) = C_bI_red'*output(1:2)';
        
        % Cap the velocities if they exceed limits
        % Checking whether our velocity is too large AND the acceleration is trying to increase said velocity... in which case we set the desired_linear_acceleration to zero.
    	% this is in the inertial frame							   
        current_velocity = [Pi_red_Vx, Pi_red_Vy, Pi_red_omega];
        
        if abs(current_velocity(1)) > VELOCITY_LIMIT(1) && sign(output(1))==sign(current_velocity(1))
            
            output(1) = 0;
            
        end
        
        if abs(current_velocity(2)) > VELOCITY_LIMIT(2) && sign(output(2))==sign(current_velocity(2))
            
            output(2) = 0;
            
        end
        
        if abs(current_velocity(3)) > VELOCITY_LIMIT(3) && sign(output(3))==sign(current_velocity(3))
            
            output(3) = 0;
            
        end
        
    end
    
    Ax_command = output(1);
    Ay_command = output(2);
    Az_command = output(3);
                             
end

== matlab function ArmDynamicsOnly/Phase #3: Experiment/Change BLACK Behavior/Sub-Phase #3 /Hough Control/MATLAB Function2 ==
  data: Oy output; z input; Ox output
function [Oy, Ox]   = C3( z )
%C3 gives the rotation matrix about the z-axis for an angle 'z'
%   z - the angle about the z-axis which you rotate
%   A - the rotation matrix

Ox = [cos(z) sin(z); -sin(z) cos(z)]*[1;0];
Oy = [cos(z) sin(z); -sin(z) cos(z)]*[0;1];
end

== matlab function ArmDynamicsOnly/Phase #3: Experiment/Change BLACK Behavior/Sub-Phase #3 /Hough Control/MATLAB Function3 ==
  data: z input; Ox output
function Ox    = C3( z )
%C3 gives the rotation matrix about the z-axis for an angle 'z'
%   z - the angle about the z-axis which you rotate
%   A - the rotation matrix

Ox = [cos(z) sin(z); -sin(z) cos(z)]*[1;0];
end

== matlab function ArmDynamicsOnly/MATLAB Function ==
  data: RED input; p_red_target output; BLACK input
function p_red_target = fcn(RED, BLACK)

    Pi_red_x = RED(1);
    Pi_red_y = RED(2);
    Pi_red_theta = RED(3);
    Pi_black_x = BLACK(1);
    Pi_black_y = BLACK(2);
    Pi_black_theta = BLACK(3); 
    
    % Define the rotation matrices for the first and second satellites
    R_red = [cos(Pi_red_theta) -sin(Pi_red_theta) 0; sin(Pi_red_theta) cos(Pi_red_theta) 0; 0 0 1];
    R_black = [cos(Pi_black_theta) -sin(Pi_black_theta) 0; sin(Pi_black_theta) cos(Pi_black_theta) 0; 0 0 1];

    % Define the offset vector for the target location
    v_target_body = [0.0743; 0.2288; 0];

    % Rotate the offset vector into the inertial frame
    v_target_inertial = R_black * v_target_body;

    % Compute the position of the center of mass of the second satellite in the inertial frame
    p_black_inertial = [Pi_black_x; Pi_black_y; 0] + v_target_inertial;

    % Compute the position of the center of mass of the second satellite in the first satellite's frame
    p_black_relative = R_red' * (p_black_inertial - [Pi_red_x; Pi_red_y; 0]);

    % Compute the position of the target in the first satellite's frame
    p_red_target = p_black_relative;
    
    % Add a bit to the x-direction for more oumph
    p_red_target(1) = p_red_target(1) + 0.07;
    p_red_target(2) = p_red_target(2) - 0.08;
   
end

== matlab function ArmDynamicsOnly/Phase #3: Experiment/Change BLACK Behavior/Sub-Phase #1/Hough Control/MATLAB Function2 ==
  data: Oy output; z input; Ox output
function [Oy, Ox]   = C3( z )
%C3 gives the rotation matrix about the z-axis for an angle 'z'
%   z - the angle about the z-axis which you rotate
%   A - the rotation matrix

Ox = [cos(z) sin(z); -sin(z) cos(z)]*[1;0];
Oy = [cos(z) sin(z); -sin(z) cos(z)]*[0;1];
end

== matlab function ArmDynamicsOnly/Phase #3: Experiment/Change BLACK Behavior/Sub-Phase #1/Hough Control/MATLAB Function3 ==
  data: z input; Ox output
function Ox    = C3( z )
%C3 gives the rotation matrix about the z-axis for an angle 'z'
%   z - the angle about the z-axis which you rotate
%   A - the rotation matrix

Ox = [cos(z) sin(z); -sin(z) cos(z)]*[1;0];
end

== matlab function ArmDynamicsOnly/Simulate Plant Dynamics/BLUE Dynamics/BLUE  Dynamics Model/MATLAB Function ==
  data: control_inputs input; x_ddot output; model_param parameter
function x_ddot = BLUE_dynamics(control_inputs, model_param)

%#codegen
% Fully define the size of x_ddot() for code generation:
x_ddot     = zeros(3,1);

% Extract the servicer model parameters from the model_param vector defined
% in initialize.m:
m_BLUE    = model_param(5);
I_BLUE    = model_param(6);

% Extract the control inputs from the control_input vector:
Fx        = control_inputs(1);              % [N]
Fy        = control_inputs(2);              % [N]
Tz        = control_inputs(3);              % [N.m]

% Calculate the state acceleration vector:
x_ddot(1) = Fx/m_BLUE;                      % [m/s^2]
x_ddot(2) = Fy/m_BLUE;                      % [m/s^2]
x_ddot(3) = Tz/I_BLUE;                      % [rad/s^2]

end

== matlab function ArmDynamicsOnly/Phase #3: Experiment/Change BLUE Behavior/Sub-Phase #4/Hough Control/MATLAB Function2 ==
  data: Oy output; z input; Ox output
function [Oy, Ox]   = C3( z )
%C3 gives the rotation matrix about the z-axis for an angle 'z'
%   z - the angle about the z-axis which you rotate
%   A - the rotation matrix

Ox = [cos(z) sin(z); -sin(z) cos(z)]*[1;0];
Oy = [cos(z) sin(z); -sin(z) cos(z)]*[0;1];
end

== matlab function ArmDynamicsOnly/Phase #3: Experiment/Change BLUE Behavior/Sub-Phase #4/Hough Control/MATLAB Function3 ==
  data: z input; Ox output
function Ox    = C3( z )
%C3 gives the rotation matrix about the z-axis for an angle 'z'
%   z - the angle about the z-axis which you rotate
%   A - the rotation matrix

Ox = [cos(z) sin(z); -sin(z) cos(z)]*[1;0];
end

== matlab function ArmDynamicsOnly/Phase #5: Hold Home/Change BLACK Behavior/Hough Control/MATLAB Function2 ==
  data: Oy output; z input; Ox output
function [Oy, Ox]   = C3( z )
%C3 gives the rotation matrix about the z-axis for an angle 'z'
%   z - the angle about the z-axis which you rotate
%   A - the rotation matrix

Ox = [cos(z) sin(z); -sin(z) cos(z)]*[1;0];
Oy = [cos(z) sin(z); -sin(z) cos(z)]*[0;1];
end
